simulink model "gm_test_min_cost_function_without_delays"  (R2022a)
settings: Solver=FixedStepDiscrete  StartTime=0.0  StopTime=10.0  RelTol=1e-3
undefined symbols (not defined in the file or in its folder): f_c
libraries: hdlmdlgenlib x80
(part 3 of 3)

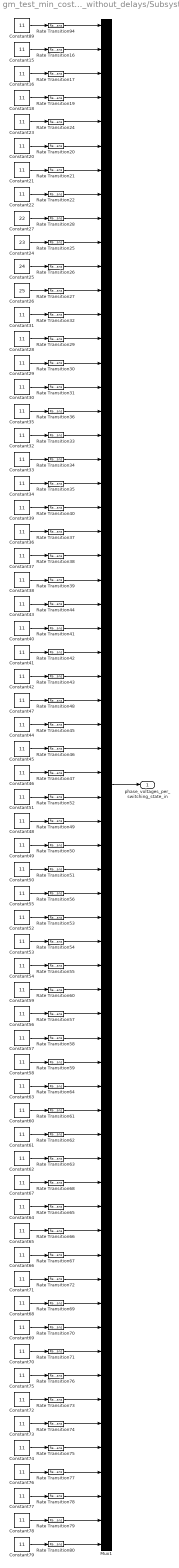
== system gm_test_min_cost_function_without_delays/Subsystem ==
  Constant{15..16,18,20..23,28..79,89} (60 alike) : Constant  Value=11  OutDataTypeStr=fixdt(1,24,11)  SampleTime=-1  LockScale=on
  Constant24 : Constant  Value=23  OutDataTypeStr=fixdt(1,24,11)  SampleTime=-1  LockScale=on
  Constant25 : Constant  Value=24  OutDataTypeStr=fixdt(1,24,11)  SampleTime=-1  LockScale=on
  Constant26 : Constant  Value=25  OutDataTypeStr=fixdt(1,24,11)  SampleTime=-1  LockScale=on
  Constant27 : Constant  Value=22  OutDataTypeStr=fixdt(1,24,11)  SampleTime=-1  LockScale=on
  Mux1 : Mux  Inputs=64
  Rate Transition{16..17,19..22,24..80,94} (64 alike) : RateTransition  OutPortSampleTime=Rt
  phase_voltages_per_switching_state_in : Outport  VectorParamsAs1DForOutWhenUnconnected=off
  wires:
  Constant59/1 -> Rate Transition60/1
  Rate Transition68/1 -> Mux1/49
  Rate Transition63/1 -> Mux1/48
  Rate Transition65/1 -> Mux1/50
  Rate Transition58/1 -> Mux1/43
  Rate Transition50/1 -> Mux1/35
  Rate Transition56/1 -> Mux1/37
  Rate Transition64/1 -> Mux1/45
  Rate Transition66/1 -> Mux1/51
  Rate Transition57/1 -> Mux1/42
  Constant39/1 -> Rate Transition40/1
  Rate Transition41/1 -> Mux1/26
  Rate Transition31/1 -> Mux1/16
  Rate Transition37/1 -> Mux1/22
  Rate Transition35/1 -> Mux1/20
  Constant73/1 -> Rate Transition74/1
  Rate Transition47/1 -> Mux1/32
  Rate Transition26/1 -> Mux1/11
  Rate Transition46/1 -> Mux1/31
  Rate Transition40/1 -> Mux1/21
  Constant74/1 -> Rate Transition75/1
  Constant79/1 -> Rate Transition80/1
  Rate Transition27/1 -> Mux1/12
  Constant57/1 -> Rate Transition58/1
  Rate Transition20/1 -> Mux1/6
  Rate Transition33/1 -> Mux1/18
  Rate Transition22/1 -> Mux1/8
  Rate Transition21/1 -> Mux1/7
  Constant78/1 -> Rate Transition79/1
  Rate Transition30/1 -> Mux1/15
  Rate Transition19/1 -> Mux1/4
  Constant38/1 -> Rate Transition39/1
  Rate Transition29/1 -> Mux1/14
  Constant76/1 -> Rate Transition77/1
  Constant72/1 -> Rate Transition73/1
  Rate Transition42/1 -> Mux1/27
  Constant65/1 -> Rate Transition66/1
  Constant64/1 -> Rate Transition65/1
  Constant71/1 -> Rate Transition72/1
  Constant53/1 -> Rate Transition54/1
  Constant69/1 -> Rate Transition70/1
  Constant40/1 -> Rate Transition41/1
  Constant63/1 -> Rate Transition64/1
  Constant60/1 -> Rate Transition61/1
  Constant77/1 -> Rate Transition78/1
  Constant25/1 -> Rate Transition26/1
  Constant26/1 -> Rate Transition27/1
  Constant62/1 -> Rate Transition63/1
  Constant52/1 -> Rate Transition53/1
  Constant49/1 -> Rate Transition50/1
  Constant16/1 -> Rate Transition17/1
  Constant45/1 -> Rate Transition46/1
  Constant58/1 -> Rate Transition59/1
  Constant23/1 -> Rate Transition24/1
  Constant51/1 -> Rate Transition52/1
  Constant44/1 -> Rate Transition45/1
  Rate Transition43/1 -> Mux1/28
  Constant89/1 -> Rate Transition94/1
  Constant50/1 -> Rate Transition51/1
  Constant31/1 -> Rate Transition32/1
  Rate Transition67/1 -> Mux1/52
  Constant15/1 -> Rate Transition16/1
  Rate Transition49/1 -> Mux1/34
  Constant55/1 -> Rate Transition56/1
  Rate Transition38/1 -> Mux1/23
  Constant30/1 -> Rate Transition31/1
  Constant67/1 -> Rate Transition68/1
  Rate Transition79/1 -> Mux1/63
  Rate Transition55/1 -> Mux1/40
  Rate Transition72/1 -> Mux1/53
  Rate Transition76/1 -> Mux1/57
  Rate Transition44/1 -> Mux1/25
  Rate Transition61/1 -> Mux1/46
  Constant28/1 -> Rate Transition29/1
  Rate Transition60/1 -> Mux1/41
  Rate Transition45/1 -> Mux1/30
  Constant21/1 -> Rate Transition21/1
  Rate Transition25/1 -> Mux1/10
  Rate Transition24/1 -> Mux1/5
  Constant46/1 -> Rate Transition47/1
  Constant29/1 -> Rate Transition30/1
  Rate Transition32/1 -> Mux1/13
  Constant22/1 -> Rate Transition22/1
  Constant33/1 -> Rate Transition34/1
  Constant47/1 -> Rate Transition48/1
  Constant68/1 -> Rate Transition69/1
  Constant27/1 -> Rate Transition28/1
  Constant41/1 -> Rate Transition42/1
  Rate Transition70/1 -> Mux1/55
  Rate Transition51/1 -> Mux1/36
  Constant54/1 -> Rate Transition55/1
  Rate Transition69/1 -> Mux1/54
  Rate Transition75/1 -> Mux1/60
  Rate Transition39/1 -> Mux1/24
  Rate Transition53/1 -> Mux1/38
  Rate Transition17/1 -> Mux1/3
  Constant34/1 -> Rate Transition35/1
  Rate Transition74/1 -> Mux1/59
  Rate Transition16/1 -> Mux1/2
  Constant66/1 -> Rate Transition67/1
  Rate Transition28/1 -> Mux1/9
  Rate Transition77/1 -> Mux1/61
  Constant70/1 -> Rate Transition71/1
  Constant20/1 -> Rate Transition20/1
  Constant43/1 -> Rate Transition44/1
  Rate Transition80/1 -> Mux1/64
  Rate Transition71/1 -> Mux1/56
  Rate Transition73/1 -> Mux1/58
  Rate Transition48/1 -> Mux1/29
  Constant37/1 -> Rate Transition38/1
  Constant75/1 -> Rate Transition76/1
  Rate Transition34/1 -> Mux1/19
  Constant36/1 -> Rate Transition37/1
  Rate Transition94/1 -> Mux1/1
  Constant18/1 -> Rate Transition19/1
  Rate Transition52/1 -> Mux1/33
  Rate Transition62/1 -> Mux1/47
  Rate Transition59/1 -> Mux1/44
  Constant32/1 -> Rate Transition33/1
  Constant24/1 -> Rate Transition25/1
  Constant48/1 -> Rate Transition49/1
  Mux1/1 -> phase_voltages_per_switching_state_in/1
  Constant42/1 -> Rate Transition43/1
  Constant61/1 -> Rate Transition62/1
  Constant35/1 -> Rate Transition36/1
  Rate Transition78/1 -> Mux1/62
  Constant56/1 -> Rate Transition57/1
  Rate Transition36/1 -> Mux1/17
  Rate Transition54/1 -> Mux1/39

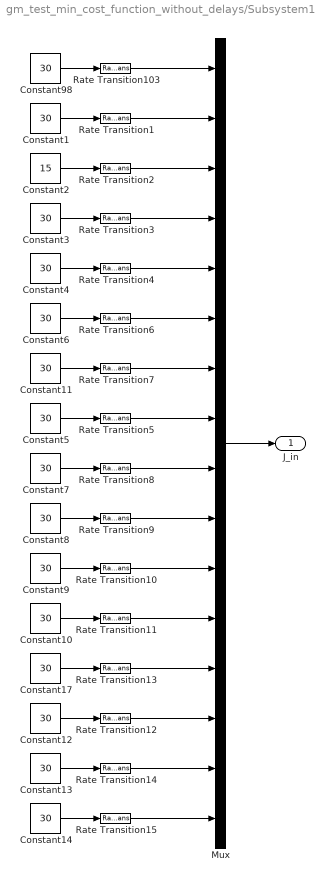
== system gm_test_min_cost_function_without_delays/Subsystem1 ==
  Constant{1,3..14,17,98} (15 alike) : Constant  Value=30  OutDataTypeStr=fixdt(1,20,11)  SampleTime=-1
  Constant2 : Constant  Value=15  OutDataTypeStr=fixdt(1,20,11)  SampleTime=-1
  Mux : Mux  Inputs=16
  Rate Transition{1..15,103} (16 alike) : RateTransition  OutPortSampleTime=Rt
  J_in : Outport
  wires:
  Mux/1 -> J_in/1
  Constant6/1 -> Rate Transition6/1
  Constant13/1 -> Rate Transition14/1
  Rate Transition11/1 -> Mux/12
  Constant8/1 -> Rate Transition9/1
  Rate Transition15/1 -> Mux/16
  Constant17/1 -> Rate Transition13/1
  Rate Transition6/1 -> Mux/6
  Constant9/1 -> Rate Transition10/1
  Constant2/1 -> Rate Transition2/1
  Constant14/1 -> Rate Transition15/1
  Constant98/1 -> Rate Transition103/1
  Rate Transition12/1 -> Mux/14
  Rate Transition8/1 -> Mux/9
  Rate Transition3/1 -> Mux/4
  Constant4/1 -> Rate Transition4/1
  Rate Transition14/1 -> Mux/15
  Rate Transition10/1 -> Mux/11
  Rate Transition7/1 -> Mux/7
  Constant10/1 -> Rate Transition11/1
  Constant7/1 -> Rate Transition8/1
  Constant5/1 -> Rate Transition5/1
  Rate Transition1/1 -> Mux/2
  Constant3/1 -> Rate Transition3/1
  Rate Transition2/1 -> Mux/3
  Constant12/1 -> Rate Transition12/1
  Rate Transition4/1 -> Mux/5
  Constant11/1 -> Rate Transition7/1
  Rate Transition5/1 -> Mux/8
  Rate Transition9/1 -> Mux/10
  Rate Transition103/1 -> Mux/1
  Rate Transition13/1 -> Mux/13
  Constant1/1 -> Rate Transition1/1

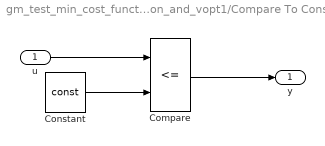
== system gm_test_min_cost_function_without_delays/Min_cost_function_and_vopt1/Compare To Constant ==
  u : Inport  OutDataTypeStr=int32  SampleTime=1e-08
  Compare : RelationalOperator  Operator=<=  OutDataTypeStr=boolean
  Constant : Constant  DisableCoverage=on  Value=const  OutDataTypeStr=Inherit: Inherit via back propagation  SampleTime=-1
  y : Outport  SampleTime=1e-08
  wires:
  u/1 -> Compare/1
  Compare/1 -> y/1
  Constant/1 -> Compare/2

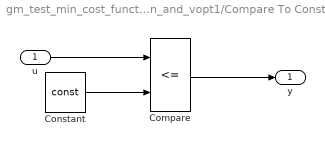
== system gm_test_min_cost_function_without_delays/Min_cost_function_and_vopt1/Compare To Constant1 ==
  u : Inport  OutDataTypeStr=fixdt(1, 33, 0)  SampleTime=1e-08
  Compare : RelationalOperator  Operator=<=  OutDataTypeStr=boolean
  Constant : Constant  DisableCoverage=on  Value=const  OutDataTypeStr=Inherit: Inherit via back propagation  SampleTime=-1
  y : Outport  SampleTime=1e-08
  wires:
  u/1 -> Compare/1
  Compare/1 -> y/1
  Constant/1 -> Compare/2

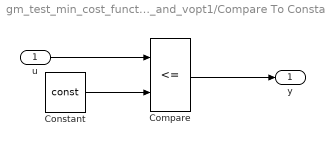
== system gm_test_min_cost_function_without_delays/Min_cost_function_and_vopt1/Compare To Constant10 ==
  u : Inport  OutDataTypeStr=fixdt(1, 33, 0)  SampleTime=1e-08
  Compare : RelationalOperator  Operator=<=  OutDataTypeStr=boolean
  Constant : Constant  DisableCoverage=on  Value=const  OutDataTypeStr=Inherit: Inherit via back propagation  SampleTime=-1
  y : Outport  SampleTime=1e-08
  wires:
  u/1 -> Compare/1
  Compare/1 -> y/1
  Constant/1 -> Compare/2

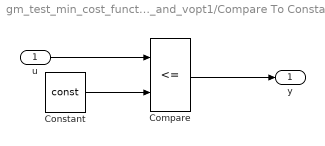
== system gm_test_min_cost_function_without_delays/Min_cost_function_and_vopt1/Compare To Constant11 ==
  u : Inport  OutDataTypeStr=fixdt(1, 33, 0)  SampleTime=1e-08
  Compare : RelationalOperator  Operator=<=  OutDataTypeStr=boolean
  Constant : Constant  DisableCoverage=on  Value=const  OutDataTypeStr=Inherit: Inherit via back propagation  SampleTime=-1
  y : Outport  SampleTime=1e-08
  wires:
  u/1 -> Compare/1
  Compare/1 -> y/1
  Constant/1 -> Compare/2

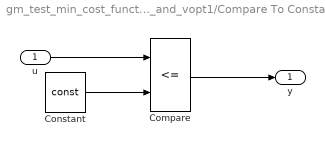
== system gm_test_min_cost_function_without_delays/Min_cost_function_and_vopt1/Compare To Constant12 ==
  u : Inport  OutDataTypeStr=fixdt(1, 33, 0)  SampleTime=1e-08
  Compare : RelationalOperator  Operator=<=  OutDataTypeStr=boolean
  Constant : Constant  DisableCoverage=on  Value=const  OutDataTypeStr=Inherit: Inherit via back propagation  SampleTime=-1
  y : Outport  SampleTime=1e-08
  wires:
  u/1 -> Compare/1
  Compare/1 -> y/1
  Constant/1 -> Compare/2

== system gm_test_min_cost_function_without_delays/Min_cost_function_and_vopt1/Compare To Constant13 ==
  u : Inport  OutDataTypeStr=fixdt(1, 33, 0)  SampleTime=1e-08
  Compare : RelationalOperator  Operator=<=  OutDataTypeStr=boolean
  Constant : Constant  DisableCoverage=on  Value=const  OutDataTypeStr=Inherit: Inherit via back propagation  SampleTime=-1
  y : Outport  SampleTime=1e-08
  wires:
  u/1 -> Compare/1
  Compare/1 -> y/1
  Constant/1 -> Compare/2

== system gm_test_min_cost_function_without_delays/Min_cost_function_and_vopt1/Compare To Constant14 ==
  u : Inport  OutDataTypeStr=fixdt(1, 33, 0)  SampleTime=1e-08
  Compare : RelationalOperator  Operator=<=  OutDataTypeStr=boolean
  Constant : Constant  DisableCoverage=on  Value=const  OutDataTypeStr=Inherit: Inherit via back propagation  SampleTime=-1
  y : Outport  SampleTime=1e-08
  wires:
  u/1 -> Compare/1
  Compare/1 -> y/1
  Constant/1 -> Compare/2

== system gm_test_min_cost_function_without_delays/Min_cost_function_and_vopt1/Compare To Constant15 ==
  u : Inport  OutDataTypeStr=fixdt(1, 33, 0)  SampleTime=1e-08
  Compare : RelationalOperator  Operator=<=  OutDataTypeStr=boolean
  Constant : Constant  DisableCoverage=on  Value=const  OutDataTypeStr=Inherit: Inherit via back propagation  SampleTime=-1
  y : Outport  SampleTime=1e-08
  wires:
  u/1 -> Compare/1
  Compare/1 -> y/1
  Constant/1 -> Compare/2

== system gm_test_min_cost_function_without_delays/Min_cost_function_and_vopt1/Compare To Constant2 ==
  u : Inport  OutDataTypeStr=fixdt(1, 33, 0)  SampleTime=1e-08
  Compare : RelationalOperator  Operator=<=  OutDataTypeStr=boolean
  Constant : Constant  DisableCoverage=on  Value=const  OutDataTypeStr=Inherit: Inherit via back propagation  SampleTime=-1
  y : Outport  SampleTime=1e-08
  wires:
  u/1 -> Compare/1
  Compare/1 -> y/1
  Constant/1 -> Compare/2

== system gm_test_min_cost_function_without_delays/Min_cost_function_and_vopt1/Compare To Constant3 ==
  u : Inport  OutDataTypeStr=fixdt(1, 33, 0)  SampleTime=1e-08
  Compare : RelationalOperator  Operator=<=  OutDataTypeStr=boolean
  Constant : Constant  DisableCoverage=on  Value=const  OutDataTypeStr=Inherit: Inherit via back propagation  SampleTime=-1
  y : Outport  SampleTime=1e-08
  wires:
  u/1 -> Compare/1
  Compare/1 -> y/1
  Constant/1 -> Compare/2

== system gm_test_min_cost_function_without_delays/Min_cost_function_and_vopt1/Compare To Constant4 ==
  u : Inport  OutDataTypeStr=fixdt(1, 33, 0)  SampleTime=1e-08
  Compare : RelationalOperator  Operator=<=  OutDataTypeStr=boolean
  Constant : Constant  DisableCoverage=on  Value=const  OutDataTypeStr=Inherit: Inherit via back propagation  SampleTime=-1
  y : Outport  SampleTime=1e-08
  wires:
  u/1 -> Compare/1
  Compare/1 -> y/1
  Constant/1 -> Compare/2

== system gm_test_min_cost_function_without_delays/Min_cost_function_and_vopt1/Compare To Constant5 ==
  u : Inport  OutDataTypeStr=fixdt(1, 33, 0)  SampleTime=1e-08
  Compare : RelationalOperator  Operator=<=  OutDataTypeStr=boolean
  Constant : Constant  DisableCoverage=on  Value=const  OutDataTypeStr=Inherit: Inherit via back propagation  SampleTime=-1
  y : Outport  SampleTime=1e-08
  wires:
  u/1 -> Compare/1
  Compare/1 -> y/1
  Constant/1 -> Compare/2

== system gm_test_min_cost_function_without_delays/Min_cost_function_and_vopt1/Compare To Constant6 ==
  u : Inport  OutDataTypeStr=fixdt(1, 33, 0)  SampleTime=1e-08
  Compare : RelationalOperator  Operator=<=  OutDataTypeStr=boolean
  Constant : Constant  DisableCoverage=on  Value=const  OutDataTypeStr=Inherit: Inherit via back propagation  SampleTime=-1
  y : Outport  SampleTime=1e-08
  wires:
  u/1 -> Compare/1
  Compare/1 -> y/1
  Constant/1 -> Compare/2

== system gm_test_min_cost_function_without_delays/Min_cost_function_and_vopt1/Compare To Constant7 ==
  u : Inport  OutDataTypeStr=fixdt(1, 33, 0)  SampleTime=1e-08
  Compare : RelationalOperator  Operator=<=  OutDataTypeStr=boolean
  Constant : Constant  DisableCoverage=on  Value=const  OutDataTypeStr=Inherit: Inherit via back propagation  SampleTime=-1
  y : Outport  SampleTime=1e-08
  wires:
  u/1 -> Compare/1
  Compare/1 -> y/1
  Constant/1 -> Compare/2

== system gm_test_min_cost_function_without_delays/Min_cost_function_and_vopt1/Compare To Constant8 ==
  u : Inport  OutDataTypeStr=fixdt(1, 33, 0)  SampleTime=1e-08
  Compare : RelationalOperator  Operator=<=  OutDataTypeStr=boolean
  Constant : Constant  DisableCoverage=on  Value=const  OutDataTypeStr=Inherit: Inherit via back propagation  SampleTime=-1
  y : Outport  SampleTime=1e-08
  wires:
  u/1 -> Compare/1
  Compare/1 -> y/1
  Constant/1 -> Compare/2

== system gm_test_min_cost_function_without_delays/Min_cost_function_and_vopt1/Compare To Constant9 ==
  u : Inport  OutDataTypeStr=fixdt(1, 33, 0)  SampleTime=1e-08
  Compare : RelationalOperator  Operator=<=  OutDataTypeStr=boolean
  Constant : Constant  DisableCoverage=on  Value=const  OutDataTypeStr=Inherit: Inherit via back propagation  SampleTime=-1
  y : Outport  SampleTime=1e-08
  wires:
  u/1 -> Compare/1
  Compare/1 -> y/1
  Constant/1 -> Compare/2

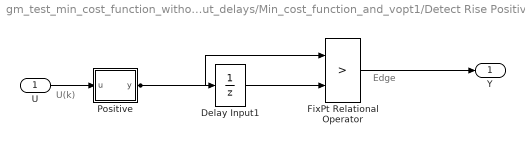
== system gm_test_min_cost_function_without_delays/Min_cost_function_and_vopt1/Detect Rise Positive ==
  note: Edge
  note: U(k)
  U : Inport  OutDataTypeStr=boolean  SampleTime=1e-08
  Delay Input1 : UnitDelay  Description=Store in Global RAM  DisableCoverage=on  InitialCondition=vinit  SampleTime=-1  HasFrameUpgradeWarning=on
  FixPt Relational Operator : RelationalOperator  Operator=>  OutDataTypeStr=boolean  ZeroCross=off  InputSameDT=off
  Positive : Subsystem  mask(Compare To Zero){relop=>, OutDataTypeStr=boolean, ZeroCross=off}
      mask prompts: relop "Simulink:masks:Operator_MP"; OutDataTypeStr "Simulink:masks:OutputDataType_MP"; ZeroCross "Simulink:masks:EnableZerocrossingDetection_MP"
      mask help: Simulink:masks:CompareToZero_MD
      mask init:
      | OutDataTypeStr = 'boolean';
      | ZeroCross = 'off';
      | blkName = 'test_min_cost_function_without_delays/Min_cost_function_and_vopt1/Detect Rise\nPositive/Positive';
      | relop = '>';
      | setValue = 'boolean';
      mask TypeOptions relop: == | ~= | < | <= | >= | >
      mask TypeOptions OutDataTypeStr: Simulink:masks:uint8 | Simulink:masks:boolean
      mask Callback ZeroCross: sl('zeroCrossEnable', gcbh);
      mask Display: disp([relop,' 0'])
  Y : Outport  SampleTime=1e-08
  wires:
  U/1 -> Positive/1(u)
  Delay Input1/1 -> FixPt Relational Operator/2
  FixPt Relational Operator/1 -> Y/1
  Positive/1(y) -> FixPt Relational Operator/1, Delay Input1/1

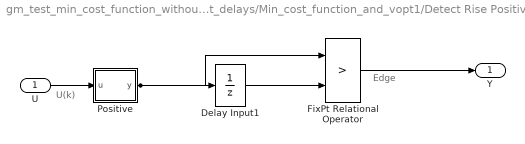
== system gm_test_min_cost_function_without_delays/Min_cost_function_and_vopt1/Detect Rise Positive1 ==
  note: Edge
  note: U(k)
  U : Inport  OutDataTypeStr=boolean  SampleTime=1e-08
  Delay Input1 : UnitDelay  Description=Store in Global RAM  DisableCoverage=on  InitialCondition=vinit  SampleTime=-1  HasFrameUpgradeWarning=on
  FixPt Relational Operator : RelationalOperator  Operator=>  OutDataTypeStr=boolean  ZeroCross=off  InputSameDT=off
  Positive : Subsystem  mask(Compare To Zero){relop=>, OutDataTypeStr=boolean, ZeroCross=off}
      mask prompts: relop "Simulink:masks:Operator_MP"; OutDataTypeStr "Simulink:masks:OutputDataType_MP"; ZeroCross "Simulink:masks:EnableZerocrossingDetection_MP"
      mask help: Simulink:masks:CompareToZero_MD
      mask init:
      | OutDataTypeStr = 'boolean';
      | ZeroCross = 'off';
      | blkName = 'test_min_cost_function_without_delays/Min_cost_function_and_vopt1/Detect Rise\nPositive1/Positive';
      | relop = '>';
      | setValue = 'boolean';
      mask TypeOptions relop: == | ~= | < | <= | >= | >
      mask TypeOptions OutDataTypeStr: Simulink:masks:uint8 | Simulink:masks:boolean
      mask Callback ZeroCross: sl('zeroCrossEnable', gcbh);
      mask Display: disp([relop,' 0'])
  Y : Outport  SampleTime=1e-08
  wires:
  U/1 -> Positive/1(u)
  Delay Input1/1 -> FixPt Relational Operator/2
  FixPt Relational Operator/1 -> Y/1
  Positive/1(y) -> FixPt Relational Operator/1, Delay Input1/1

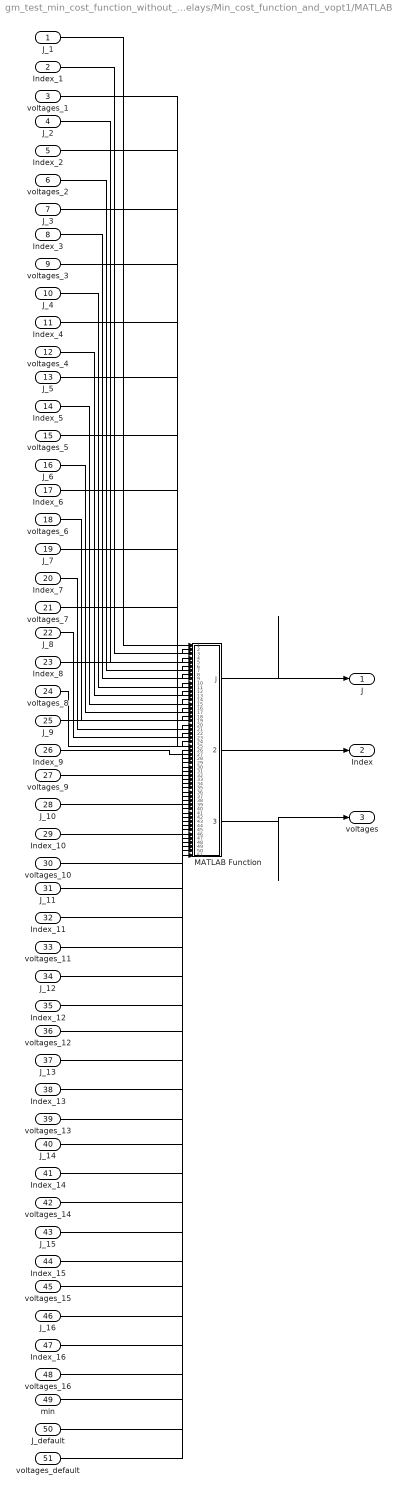
== system gm_test_min_cost_function_without_delays/Min_cost_function_and_vopt1/MATLAB Function ==
  J_1 : Inport  OutDataTypeStr=fixdt(1, 20, 11)  PortDimensions=1  SampleTime=1e-08
  Index_1 : Inport  Port=2  OutDataTypeStr=int32  PortDimensions=1  SampleTime=1e-08
  voltages_1 : Inport  Port=3  OutDataTypeStr=fixdt(1, 24, 11)  PortDimensions=[4]  SampleTime=1e-08
  J_2 : Inport  Port=4  OutDataTypeStr=fixdt(1, 20, 11)  PortDimensions=1  SampleTime=1e-08
  Index_2 : Inport  Port=5  OutDataTypeStr=int32  PortDimensions=1  SampleTime=1e-08
  voltages_2 : Inport  Port=6  OutDataTypeStr=fixdt(1, 24, 11)  PortDimensions=[4]  SampleTime=1e-08
  J_3 : Inport  Port=7  OutDataTypeStr=fixdt(1, 20, 11)  PortDimensions=1  SampleTime=1e-08
  Index_3 : Inport  Port=8  OutDataTypeStr=int32  PortDimensions=1  SampleTime=1e-08
  voltages_3 : Inport  Port=9  OutDataTypeStr=fixdt(1, 24, 11)  PortDimensions=[4]  SampleTime=1e-08
  J_4 : Inport  Port=10  OutDataTypeStr=fixdt(1, 20, 11)  PortDimensions=1  SampleTime=1e-08
  Index_4 : Inport  Port=11  OutDataTypeStr=int32  PortDimensions=1  SampleTime=1e-08
  voltages_4 : Inport  Port=12  OutDataTypeStr=fixdt(1, 24, 11)  PortDimensions=[4]  SampleTime=1e-08
  J_5 : Inport  Port=13  OutDataTypeStr=fixdt(1, 20, 11)  PortDimensions=1  SampleTime=1e-08
  Index_5 : Inport  Port=14  OutDataTypeStr=int32  PortDimensions=1  SampleTime=1e-08
  voltages_5 : Inport  Port=15  OutDataTypeStr=fixdt(1, 24, 11)  PortDimensions=[4]  SampleTime=1e-08
  J_6 : Inport  Port=16  OutDataTypeStr=fixdt(1, 20, 11)  PortDimensions=1  SampleTime=1e-08
  Index_6 : Inport  Port=17  OutDataTypeStr=int32  PortDimensions=1  SampleTime=1e-08
  voltages_6 : Inport  Port=18  OutDataTypeStr=fixdt(1, 24, 11)  PortDimensions=[4]  SampleTime=1e-08
  J_7 : Inport  Port=19  OutDataTypeStr=fixdt(1, 20, 11)  PortDimensions=1  SampleTime=1e-08
  Index_7 : Inport  Port=20  OutDataTypeStr=int32  PortDimensions=1  SampleTime=1e-08
  voltages_7 : Inport  Port=21  OutDataTypeStr=fixdt(1, 24, 11)  PortDimensions=[4]  SampleTime=1e-08
  J_8 : Inport  Port=22  OutDataTypeStr=fixdt(1, 20, 11)  PortDimensions=1  SampleTime=1e-08
  Index_8 : Inport  Port=23  OutDataTypeStr=int32  PortDimensions=1  SampleTime=1e-08
  voltages_8 : Inport  Port=24  OutDataTypeStr=fixdt(1, 24, 11)  PortDimensions=[4]  SampleTime=1e-08
  J_9 : Inport  Port=25  OutDataTypeStr=fixdt(1, 20, 11)  PortDimensions=1  SampleTime=1e-08
  Index_9 : Inport  Port=26  OutDataTypeStr=int32  PortDimensions=1  SampleTime=1e-08
  voltages_9 : Inport  Port=27  OutDataTypeStr=fixdt(1, 24, 11)  PortDimensions=[4]  SampleTime=1e-08
  J_10 : Inport  Port=28  OutDataTypeStr=fixdt(1, 20, 11)  PortDimensions=1  SampleTime=1e-08
  Index_10 : Inport  Port=29  OutDataTypeStr=int32  PortDimensions=1  SampleTime=1e-08
  voltages_10 : Inport  Port=30  OutDataTypeStr=fixdt(1, 24, 11)  PortDimensions=[4]  SampleTime=1e-08
  J_11 : Inport  Port=31  OutDataTypeStr=fixdt(1, 20, 11)  PortDimensions=1  SampleTime=1e-08
  Index_11 : Inport  Port=32  OutDataTypeStr=int32  PortDimensions=1  SampleTime=1e-08
  voltages_11 : Inport  Port=33  OutDataTypeStr=fixdt(1, 24, 11)  PortDimensions=[4]  SampleTime=1e-08
  J_12 : Inport  Port=34  OutDataTypeStr=fixdt(1, 20, 11)  PortDimensions=1  SampleTime=1e-08
  Index_12 : Inport  Port=35  OutDataTypeStr=int32  PortDimensions=1  SampleTime=1e-08
  voltages_12 : Inport  Port=36  OutDataTypeStr=fixdt(1, 24, 11)  PortDimensions=[4]  SampleTime=1e-08
  J_13 : Inport  Port=37  OutDataTypeStr=fixdt(1, 20, 11)  PortDimensions=1  SampleTime=1e-08
  Index_13 : Inport  Port=38  OutDataTypeStr=int32  PortDimensions=1  SampleTime=1e-08
  voltages_13 : Inport  Port=39  OutDataTypeStr=fixdt(1, 24, 11)  PortDimensions=[4]  SampleTime=1e-08
  J_14 : Inport  Port=40  OutDataTypeStr=fixdt(1, 20, 11)  PortDimensions=1  SampleTime=1e-08
  Index_14 : Inport  Port=41  OutDataTypeStr=int32  PortDimensions=1  SampleTime=1e-08
  voltages_14 : Inport  Port=42  OutDataTypeStr=fixdt(1, 24, 11)  PortDimensions=[4]  SampleTime=1e-08
  J_15 : Inport  Port=43  OutDataTypeStr=fixdt(1, 20, 11)  PortDimensions=1  SampleTime=1e-08
  Index_15 : Inport  Port=44  OutDataTypeStr=int32  PortDimensions=1  SampleTime=1e-08
  voltages_15 : Inport  Port=45  OutDataTypeStr=fixdt(1, 24, 11)  PortDimensions=[4]  SampleTime=1e-08
  J_16 : Inport  Port=46  OutDataTypeStr=fixdt(1, 20, 11)  PortDimensions=1  SampleTime=1e-08
  Index_16 : Inport  Port=47  OutDataTypeStr=int32  PortDimensions=1  SampleTime=1e-08
  voltages_16 : Inport  Port=48  OutDataTypeStr=fixdt(1, 24, 11)  PortDimensions=[4]  SampleTime=1e-08
  min : Inport  Port=49  OutDataTypeStr=fixdt(1, 20, 11)  PortDimensions=1  SampleTime=1e-08
  J_default : Inport  Port=50  OutDataTypeStr=fixdt(1, 20, 11)  PortDimensions=1  SampleTime=1e-08
  voltages_default : Inport  Port=51  OutDataTypeStr=fixdt(1, 24, 11)  PortDimensions=[4]  SampleTime=1e-08
  MATLAB Function : MATLAB Function  TreatAsAtomicUnit=on
  J : Outport  SampleTime=1e-08  VectorParamsAs1DForOutWhenUnconnected=off
  Index : Outport  Port=2  SampleTime=1e-08
  voltages : Outport  Port=3  SampleTime=1e-08
  wires:
  J_1/1 -> MATLAB Function/1(J_1)
  Index_1/1 -> MATLAB Function/2(Index_1)
  voltages_1/1 -> MATLAB Function/3(voltages_1)
  J_2/1 -> MATLAB Function/4(J_2)
  Index_2/1 -> MATLAB Function/5(Index_2)
  voltages_2/1 -> MATLAB Function/6(voltages_2)
  J_3/1 -> MATLAB Function/7(J_3)
  Index_3/1 -> MATLAB Function/8(Index_3)
  voltages_3/1 -> MATLAB Function/9(voltages_3)
  J_4/1 -> MATLAB Function/10(J_4)
  Index_4/1 -> MATLAB Function/11(Index_4)
  voltages_4/1 -> MATLAB Function/12(voltages_4)
  J_5/1 -> MATLAB Function/13(J_5)
  Index_5/1 -> MATLAB Function/14(Index_5)
  voltages_5/1 -> MATLAB Function/15(voltages_5)
  J_6/1 -> MATLAB Function/16(J_6)
  Index_6/1 -> MATLAB Function/17(Index_6)
  voltages_6/1 -> MATLAB Function/18(voltages_6)
  J_7/1 -> MATLAB Function/19(J_7)
  Index_7/1 -> MATLAB Function/20(Index_7)
  voltages_7/1 -> MATLAB Function/21(voltages_7)
  J_8/1 -> MATLAB Function/22(J_8)
  Index_8/1 -> MATLAB Function/23(Index_8)
  voltages_8/1 -> MATLAB Function/24(voltages_8)
  J_9/1 -> MATLAB Function/25(J_9)
  Index_9/1 -> MATLAB Function/26(Index_9)
  voltages_9/1 -> MATLAB Function/27(voltages_9)
  J_10/1 -> MATLAB Function/28(J_10)
  Index_10/1 -> MATLAB Function/29(Index_10)
  voltages_10/1 -> MATLAB Function/30(voltages_10)
  J_11/1 -> MATLAB Function/31(J_11)
  Index_11/1 -> MATLAB Function/32(Index_11)
  voltages_11/1 -> MATLAB Function/33(voltages_11)
  J_12/1 -> MATLAB Function/34(J_12)
  Index_12/1 -> MATLAB Function/35(Index_12)
  voltages_12/1 -> MATLAB Function/36(voltages_12)
  J_13/1 -> MATLAB Function/37(J_13)
  Index_13/1 -> MATLAB Function/38(Index_13)
  voltages_13/1 -> MATLAB Function/39(voltages_13)
  J_14/1 -> MATLAB Function/40(J_14)
  Index_14/1 -> MATLAB Function/41(Index_14)
  voltages_14/1 -> MATLAB Function/42(voltages_14)
  J_15/1 -> MATLAB Function/43(J_15)
  Index_15/1 -> MATLAB Function/44(Index_15)
  voltages_15/1 -> MATLAB Function/45(voltages_15)
  J_16/1 -> MATLAB Function/46(J_16)
  Index_16/1 -> MATLAB Function/47(Index_16)
  voltages_16/1 -> MATLAB Function/48(voltages_16)
  min/1 -> MATLAB Function/49(min)
  J_default/1 -> MATLAB Function/50(J_default)
  voltages_default/1 -> MATLAB Function/51(voltages_default)
  MATLAB Function/1(J) -> J/1
  MATLAB Function/2(Index) -> Index/1
  MATLAB Function/3(voltages) -> voltages/1

== system gm_test_min_cost_function_without_delays/Min_cost_function_and_vopt1/Detect Rise Positive/Positive ==
  u : Inport  OutDataTypeStr=boolean  SampleTime=1e-08
  Compare : RelationalOperator  Operator=>  OutDataTypeStr=boolean  ZeroCross=off
  Constant : Constant  DisableCoverage=on  Value=0  OutDataTypeStr=Inherit: Inherit via back propagation  SampleTime=-1  PreserveConstantTs=on
  y : Outport  SampleTime=1e-08
  wires:
  u/1 -> Compare/1
  Compare/1 -> y/1
  Constant/1 -> Compare/2

== system gm_test_min_cost_function_without_delays/Min_cost_function_and_vopt1/Detect Rise Positive1/Positive ==
  u : Inport  OutDataTypeStr=boolean  SampleTime=1e-08
  Compare : RelationalOperator  Operator=>  OutDataTypeStr=boolean  ZeroCross=off
  Constant : Constant  DisableCoverage=on  Value=0  OutDataTypeStr=Inherit: Inherit via back propagation  SampleTime=-1  PreserveConstantTs=on
  y : Outport  SampleTime=1e-08
  wires:
  u/1 -> Compare/1
  Compare/1 -> y/1
  Constant/1 -> Compare/2

== matlab function gm_test_min_cost_function_without_delays/Min_cost_function_and_vopt1/MATLAB Function/MATLAB Function ==
  data: J_1 input; Index_1 input; J output fixdt(1,20,11); voltages_1 input; J_2 input; Index_2 input; voltages_2 input; J_3 input; Index_3 input; voltages_3 input; J_4 input; Index_4 input; voltages_4 input; J_5 input; Index_5 input; voltages_5 input; J_6 input; Index_6 input; voltages_6 input; J_7 input; Index_7 input; voltages_7 input; J_8 input; Index_8 input; voltages_8 input; J_9 input; Index_9 input; voltages_9 input; J_10 input; Index_10 input; voltages_10 input; J_11 input; Index_11 input; voltages_11 input; J_12 input; Index_12 input; voltages_12 input; J_13 input; Index_13 input; voltages_13 input; J_14 input; Index_14 input; voltages_14 input; J_15 input; Index_15 input; voltages_15 input; J_16 input; Index_16 input; voltages_16 input; Index output int32; min input fixdt(1,20,11); J_default input; voltages output; voltages_default input
function [J, Index, voltages] = fcn(J_1, Index_1, voltages_1, J_2, Index_2, voltages_2, J_3, Index_3, voltages_3, J_4, Index_4, voltages_4, J_5, Index_5, voltages_5, J_6, Index_6, voltages_6, ...
                                    J_7, Index_7, voltages_7, J_8, Index_8, voltages_8, J_9, Index_9, voltages_9, J_10, Index_10, voltages_10, J_11, Index_11, voltages_11, J_12, Index_12, voltages_12, ...
                                    J_13, Index_13, voltages_13, J_14, Index_14, voltages_14, J_15, Index_15, voltages_15, J_16, Index_16, voltages_16, min, J_default,voltages_default)



if J_1 == min
    Index = Index_1;
    voltages = voltages_1;
    J = J_1;
elseif J_2 == min
    Index = Index_2;
    voltages = voltages_2;
    J = J_2;
elseif J_3 == min
    Index = Index_3;
    voltages = voltages_3;
    J = J_3;
elseif J_4 == min
    Index = Index_4;
    voltages = voltages_4;
    J = J_4;
elseif J_5 == min
    Index = Index_5;
    voltages = voltages_5;
    J = J_5;
elseif J_6 == min
    Index = Index_6;
    voltages = voltages_6;
    J = J_6;
elseif J_7 == min
    Index = Index_7;
    voltages = voltages_7;
    J = J_7;
elseif J_8 == min
    Index = Index_8;
    voltages = voltages_8;
    J = J_8;
elseif J_9 == min
    Index = Index_9;
    voltages = voltages_9;
    J = J_9;
elseif J_10 == min
    Index = Index_10;
    voltages = voltages_10;
    J = J_10;
elseif J_11 == min
    Index = Index_11;
    voltages = voltages_11;
    J = J_11;
elseif J_12 == min
    Index = Index_12;
    voltages = voltages_12;
    J = J_12;
elseif J_13 == min
    Index = Index_13;
    voltages = voltages_13;
    J = J_13;
elseif J_14 == min
    Index = Index_14;
    voltages = voltages_14;
    J = J_14;
elseif J_15 == min
    Index = Index_15;
    voltages = voltages_15;
    J = J_15;
elseif J_16 == min
    Index = Index_16;
    voltages = voltages_16;
    J = J_16;
else 
    Index = int32(0);
    J = J_default;
    voltages = voltages_default;
end
